simulink model "TestGroup_OLD"  (R2024b)
settings: Solver=VariableStepAuto  StartTime=0.0  StopTime=60  RelTol=1e-3
undefined symbols (not defined in the file or in its folder): A, B, C, D, UNTUNED_K
settings Model: Creator=hazza  LastModifiedBy=hazza

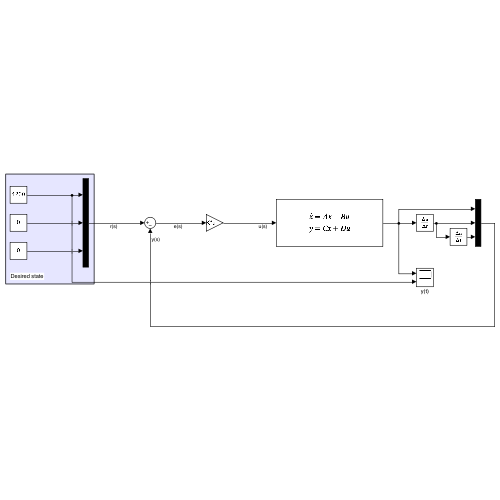
[thumbnail: Simulink's stored preview of the top-level diagram]
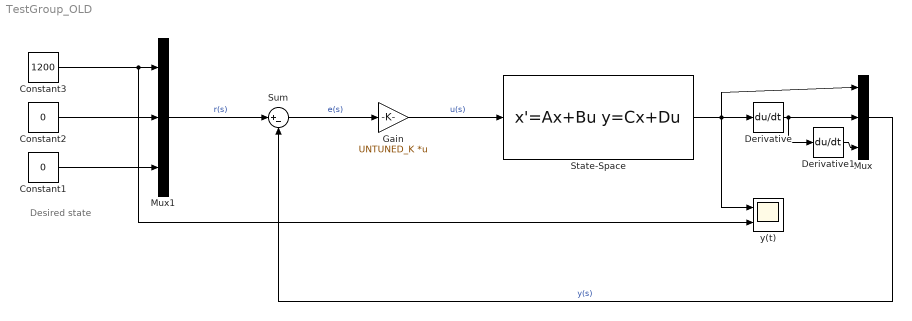
== system TestGroup_OLD ==
  note: Desired state
  Constant1 : Constant  Value=0
  Constant2 : Constant  Value=0
  Constant3 : Constant  Value=1200
  Derivative : Derivative
  Derivative1 : Derivative
  Gain : Gain  Gain=UNTUNED_K  Multiplication=Matrix(K*u)
  Mux : Mux  Inputs=3
  Mux1 : Mux  Inputs=3
  State-Space : StateSpace  A=A  B=B  C=C  D=D  InitialCondition=[1200, 0, 0]
  Sum : Sum  Inputs=|+-
  y(t) : Scope  NumInputPorts=2
  wires:
  State-Space/1 -> y(t)/1, Mux/1, Derivative/1
  Derivative/1 -> Derivative1/1, Mux/2
  Derivative1/1 -> Mux/3
  Sum/1 -> Gain/1  "e(s)"
  Gain/1 -> State-Space/1  "u(s)"
  Mux/1 -> Sum/2  "y(s)"
  Constant3/1 -> y(t)/2, Mux1/1
  Mux1/1 -> Sum/1  "r(s)"
  Constant2/1 -> Mux1/2
  Constant1/1 -> Mux1/3
